simulink model "UUV_sim"  (Simulink 8.3)
settings: Solver=ode45  StartTime=0.0  StopTime=100  RelTol=1e-3
undefined symbols (not defined in the file or in its folder): drawUUV, P, UUV_ctrl
libraries: simulink x1
settings Model: Creator=beard  LastModifiedBy=jhl48
settings OptimizationCC: ExpressionDepthLimit=2147483647  InitFltsAndDblsToZero=on
settings DebuggingCC: FcnCallInpInsideContextMsg=UseLocalSettings

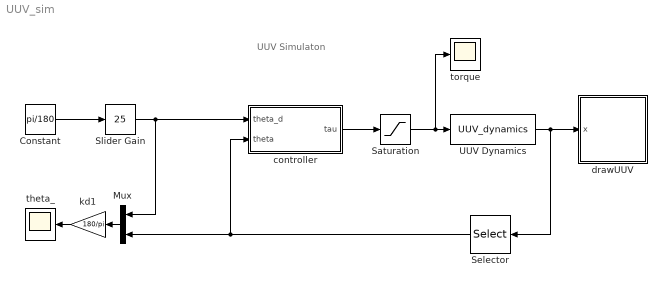
== system UUV_sim ==
  note: UUV Simulaton
  Constant : Constant  Value=pi/180
  Mux : Mux  Inputs=2
  Saturation : Saturate  UpperLimit=P.tau_max  LowerLimit=-P.tau_max
  Selector : Selector  InputPortWidth=2  Indices=[1]
  Slider Gain : simulink/Math Operations/Slider Gain  low=-180  gain=25  high=180
  UUV Dynamics : S-Function  FunctionName=UUV_dynamics  Parameters=P  EnableBusSupport=off
  controller : Subsystem
  drawUUV : Subsystem
      mask init:
      | % drawing parameters
      | MajorAxis = 10;
      | MinorAxis = 6;
      | C_M = [0;-4];
      mask Display: image(imread('tv.jpg'))
  kd1 : Gain  Gain=180/pi
  theta_ : Scope
      settings: YMin=15  YMax=15
  torque : Scope
      settings: YMin=5.55112e-17  YMax=1
  wires:
  UUV Dynamics/1 -> drawUUV/1(x), Selector/1
  Saturation/1 -> UUV Dynamics/1, torque/1
  Mux/1 -> kd1/1
  kd1/1 -> theta_/1
  controller/1(tau) -> Saturation/1
  Constant/1 -> Slider Gain/1
  Slider Gain/1 -> Mux/1, controller/1(theta_d)
  Selector/1 -> Mux/2, controller/2(theta)

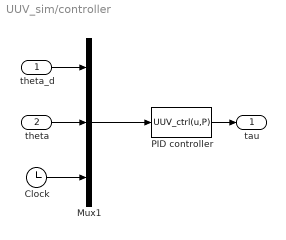
== system UUV_sim/controller ==
  theta_d : Inport
  theta : Inport  Port=2
  Clock : Clock
  Mux1 : Mux  Inputs=3
  PID controller : MATLABFcn  MATLABFcn=UUV_ctrl(u,P)  OutputDimensions=1  SampleTime=P.Ts
  tau : Outport
  wires:
  Mux1/1 -> PID controller/1
  theta_d/1 -> Mux1/1
  theta/1 -> Mux1/2
  PID controller/1 -> tau/1
  Clock/1 -> Mux1/3

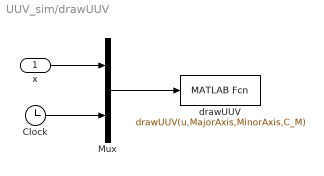
== system UUV_sim/drawUUV ==
  x : Inport
  Clock : Clock
  Mux : Mux  Inputs=2
  drawUUV : MATLABFcn  MATLABFcn=drawUUV(u,MajorAxis,MinorAxis,C_M)  OutputDimensions=0  SampleTime=0.1
  wires:
  Mux/1 -> drawUUV/1
  x/1 -> Mux/1
  Clock/1 -> Mux/2
